simulink model "OscOnly"  (R2022b)
settings: Solver=VariableStepAuto  StartTime=0.0  StopTime=1  RelTol=1e-3
libraries: simulink x1
settings Model: Creator=yoni  LastModifiedBy=yoni

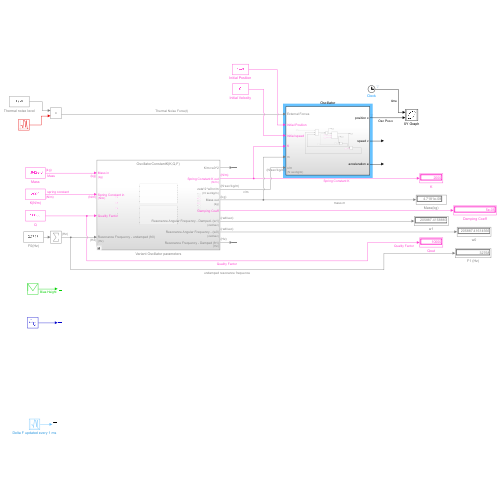
[thumbnail: Simulink's stored preview of the top-level diagram]
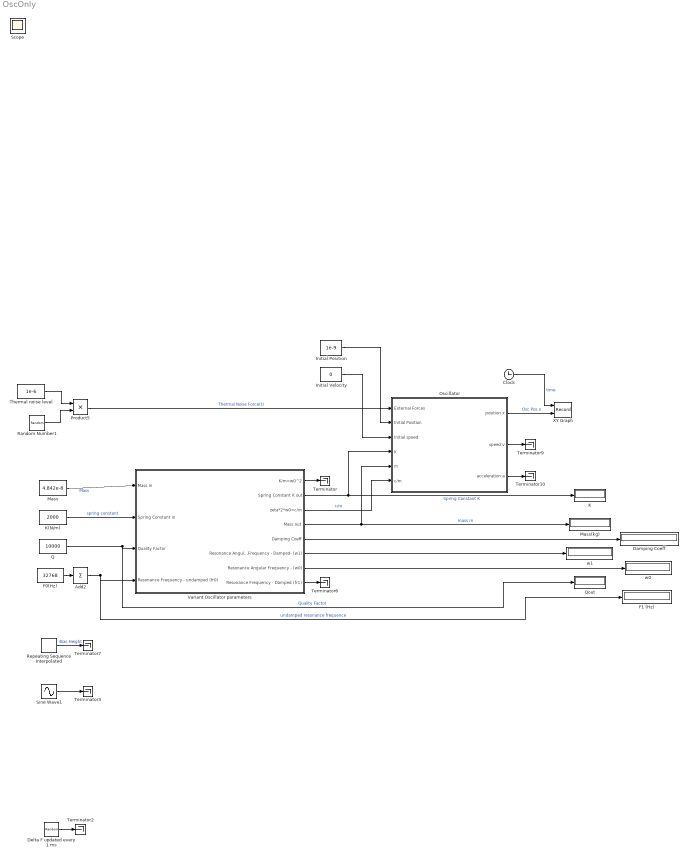
== system OscOnly ==
  Add2 : Sum  Inputs=+
  Clock : Clock
  Damping Coeff : Display
  Delta F updated every 1 ms : RandomNumber  Variance=100  Seed=7546745  SampleTime=1e-3
  F0(Hz) : Constant  Value=32768  SampleTime=-1
  F1 (Hz) : Display
  Initial Position : Constant  Value=1e-9  VectorParams1D=off
  Initial Velocity : Constant  Value=0
  K : Display
  K(N/m) : Constant  Value=2000
  Mass : Constant  Value=4.842e-8
  Mass(kg) : Display
      settings: Format=short_e
  Oscillator : Subsystem
  Product5 : Product
  Q : Constant  Value=10000
  Qout : Display
  Random Number1 : RandomNumber  Seed=4582  SampleTime=10^-8
  Repeating Sequence Interpolated : simulink/Sources/Repeating Sequence Interpolated  OutValues="[25e-10  0.6e-9 25e-10].'"  TimeValues=[0e-3 300e-3 600e-3 ].'  LookUpMeth=Interpolation-Use End Values  tsamp=1e-6  OutMin=[]  OutMax=[]  OutDataTypeStr=double  OutputDataTypeScalingMode=double  OutDataType=fixdt(0,8)  OutScaling=2^-10
  Sine Wave1 : Sin  Amplitude=20  Frequency=5000  Phase=0.0001  SampleTime=10e-6
  Terminator{,2..3,6..7,9..10} (7 alike) : Terminator
  Thermal noise level : Constant  Value=1e-6  VectorParams1D=off  SampleTime=-1
  Variant Oscillator parameters : Subsystem  Variant=on  VariantControlMode=label  LabelModeActiveChoice=OscillatorTypeVar==0  PropagateVariantConditions=on
  XY Graph : Record  FileSettingsInternal="{\"entries\":[{\"content\":{\"excelSettings\":{\"content\":{},\"type\":\"Streamout.ExcelSettings\"}},\"type\":\"Streamout.FileSettingStorage\",\"uuid\":\"efa23a6c-4987-48e8-b3f0-6b34ea382b02\"}],\"packageUris\":[\"http://schema.mathworks.com/mf0/streamout_blocks/R2020a\"],\"version\":\"1.0\"}"  Layout=[1 1]  SignalsInternal="{\"entries\":[{\"content\":{\"signals\":[{\"content\":{\"blockPath\":[\"OscOnly/XY Graph\"],\"channel\":[],\"dimensions\":[1],\"domain\":\"OscOnly/XY Graph\",\"lineColor\":\"#a2142f\",\"plots\":[1],\"port\":1,\"sid\":[\"\"],\"signalID\":691948,\"signalName\":\"time\"},\"type\":\"RecordBlkView.Signal\",\"uuid\":\"d217d77e-fb47-4b7d-b3a2-eb88acfcbc3e\"},{\"content\":{\"blockPath\":[\"OscOnly/XY Graph\"],\"channel\":[],\"dimensions\":[1],\"domain\":\"OscOnly/XY Graph\",\"lineColor\":\"#139fff\",\"plots\":[1],\"port\":2,\"sid\":[\"\"],\"signalID\":691952,\"signalName\":\"Osc Pos x\"},\"type\":\"RecordBlkView.Signal\",\"uuid\":\"5dfddc15-8547-4e19-ad7f-01361fb84854\"}]},\"type\":\"RecordBlkView.InputSignals\",\"uuid\":\"3171f09f-039c-4b49-abe8-6842aea79503\"}],\"packageUris\":[\"http://schema.mathworks.com/mf0/streamout_blocks/R2020a\"],\"version\":\"1.0\"}"  VisualizationBindings="{\"xyplotplugin\":{\"info\":[{\"series\":[{\"bindingParametersList\":[{\"parameter\":\"X-Axis\",\"signalID\":691948,\"signalName\":\"time\"},{\"parameter\":\"Y-Axis\",\"signalID\":691952,\"signalName\":\"Osc Pos x\"}],\"seriesID\":49762}],\"subplotID\":1}]}}"  CompatibilityTag=XY
  w0 : Display
  w1 : Display
  Scope : Scope
  wires:
  Oscillator/2(speed v) -> Terminator9/1
  Initial Velocity/1 -> Oscillator/3(Initial speed)
  Product5/1 -> Oscillator/1(External Forces)  "Thermal Noise Force(t)"
  Variant Oscillator parameters/7(Resonance Angular Frequency - (w0)) -> w0/1
  Oscillator/3(acceleration a) -> Terminator10/1
  Add2/1 -> Variant Oscillator parameters/4(Resonance Frequency - undamped (fr0)), F1 (Hz)/1  "undamped resonance frequence"
  Q/1 -> Variant Oscillator parameters/3(Quality Factor), Qout/1  "Quality Factor"
  Delta F updated every 1 ms/1 -> Terminator2/1
  Variant Oscillator parameters/8(Resonance Frequency - Damped (fr1)) -> Terminator6/1
  Variant Oscillator parameters/6(Resonance Angular Frequency - Damped- (w1)) -> w1/1
  Random Number1/1 -> Product5/2
  Thermal noise level/1 -> Product5/1
  Initial Position/1 -> Oscillator/2(Initial Position)
  Variant Oscillator parameters/3(zeta*2*w0=c/m) -> Oscillator/6(c/m)  "c/m"
  Repeating Sequence Interpolated/1 -> Terminator7/1  "Bias Height"
  Mass/1 -> Variant Oscillator parameters/1(Mass in)  "Mass"
  Variant Oscillator parameters/2(Spring Constant K out) -> K/1, Oscillator/4(K)  "Spring Constant K"
  F0(Hz)/1 -> Add2/1
  Variant Oscillator parameters/4(Mass out) -> Mass(kg)/1, Oscillator/5(m)  "mass m"
  K(N/m)/1 -> Variant Oscillator parameters/2(Spring Constant in)  "spring constant"
  Variant Oscillator parameters/1(K/m=w0^2) -> Terminator/1
  Variant Oscillator parameters/5(Damping Coeff) -> Damping Coeff/1
  Sine Wave1/1 -> Terminator3/1
  Oscillator/1(" position x") -> XY Graph/2  "Osc Pos x"
  Clock/1 -> XY Graph/1  "time"

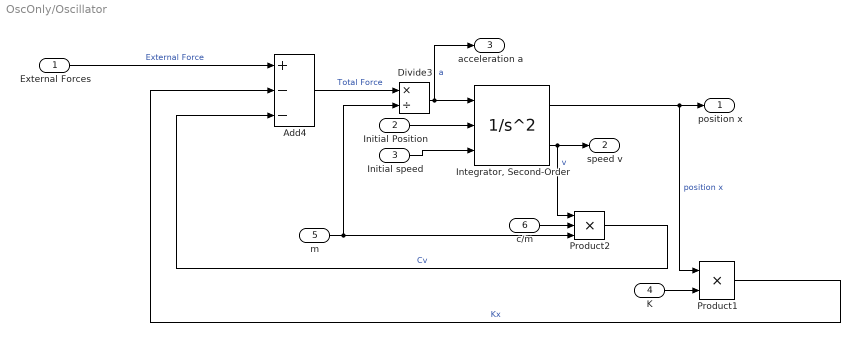
== system OscOnly/Oscillator ==
  External Forces : Inport
  Initial Position : Inport  Port=2
  Initial speed : Inport  Port=3
  K : Inport  Port=4
  m : Inport  Port=5
  c/m : Inport  Port=6  Unit=N*sec/kg/m
  Add4 : Sum  Inputs=+--
  Divide3 : Product  Inputs=*/
  "Integrator, Second-Order" : SecondOrderIntegrator  ICSourceX=external  LimitX=on  UpperLimitX=0.01  LowerLimitX=-0.01  ICSourceDXDT=external
  Product1 : Product
  Product2 : Product  Inputs=3
  " position x" : Outport
  speed v : Outport  Port=2
  acceleration a : Outport  Port=3
  wires:
  Divide3/1 -> "Integrator, Second-Order"/1, acceleration a/1  "a"
  m/1 -> Divide3/2, Product2/3
  Product1/1 -> Add4/2  "Kx"
  c/m/1 -> Product2/2
  Initial speed/1 -> "Integrator, Second-Order"/3
  Add4/1 -> Divide3/1  "Total Force"
  External Forces/1 -> Add4/1  "External Force"
  K/1 -> Product1/2
  "Integrator, Second-Order"/2 -> speed v/1, Product2/1  "v"
  Product2/1 -> Add4/3  "Cv"
  "Integrator, Second-Order"/1 -> Product1/1, " position x"/1  "position x"
  Initial Position/1 -> "Integrator, Second-Order"/2

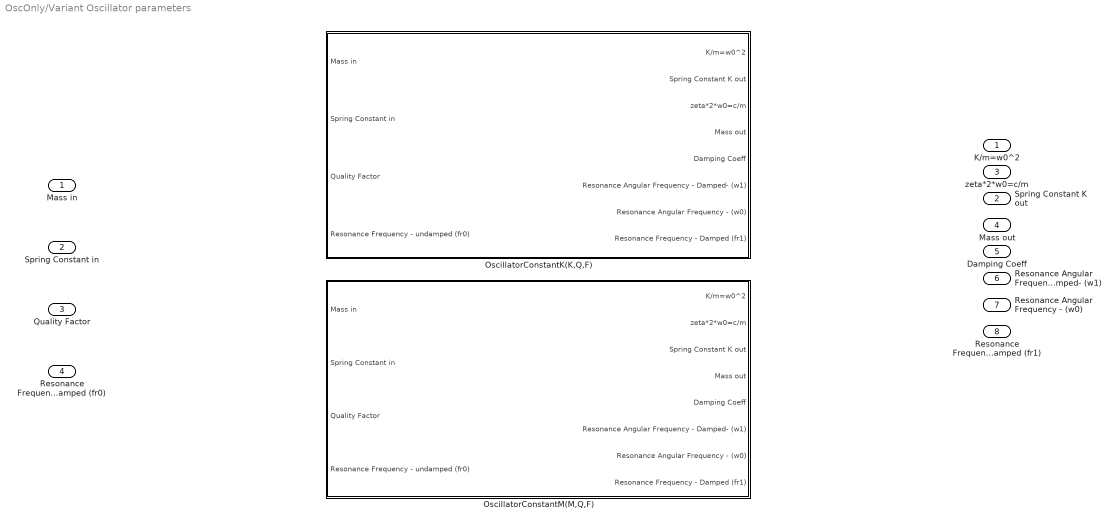
== system OscOnly/Variant Oscillator parameters ==
  Mass in : Inport  Unit=kg
  Spring Constant in : Inport  Port=2  Unit=N/m
  Quality Factor : Inport  Port=3
  Resonance Frequency - undamped (fr0) : Inport  Port=4  Unit=Hz
  OscillatorConstantK(K,Q,F) : Subsystem  VariantControl=OscillatorTypeVar==0
  OscillatorConstantM(M,Q,F) : Subsystem  VariantControl=OscillatorTypeVar==1
  K/m=w0^2 : Outport  VectorParamsAs1DForOutWhenUnconnected=off
  Spring Constant K out : Outport  Port=2  Unit=N/m  VectorParamsAs1DForOutWhenUnconnected=off
  zeta*2*w0=c/m : Outport  Port=3  Unit=N*sec/kg/m  VectorParamsAs1DForOutWhenUnconnected=off
  Mass out : Outport  Port=4  Unit=kg  VectorParamsAs1DForOutWhenUnconnected=off
  Damping Coeff : Outport  Port=5  VectorParamsAs1DForOutWhenUnconnected=off
  Resonance Angular Frequency - Damped- (w1) : Outport  Port=6  Unit=rad/sec  VectorParamsAs1DForOutWhenUnconnected=off
  Resonance Angular Frequency - (w0) : Outport  Port=7  Unit=rad/sec  VectorParamsAs1DForOutWhenUnconnected=off
  Resonance Frequency - Damped (fr1) : Outport  Port=8  Unit=Hz  VectorParamsAs1DForOutWhenUnconnected=off

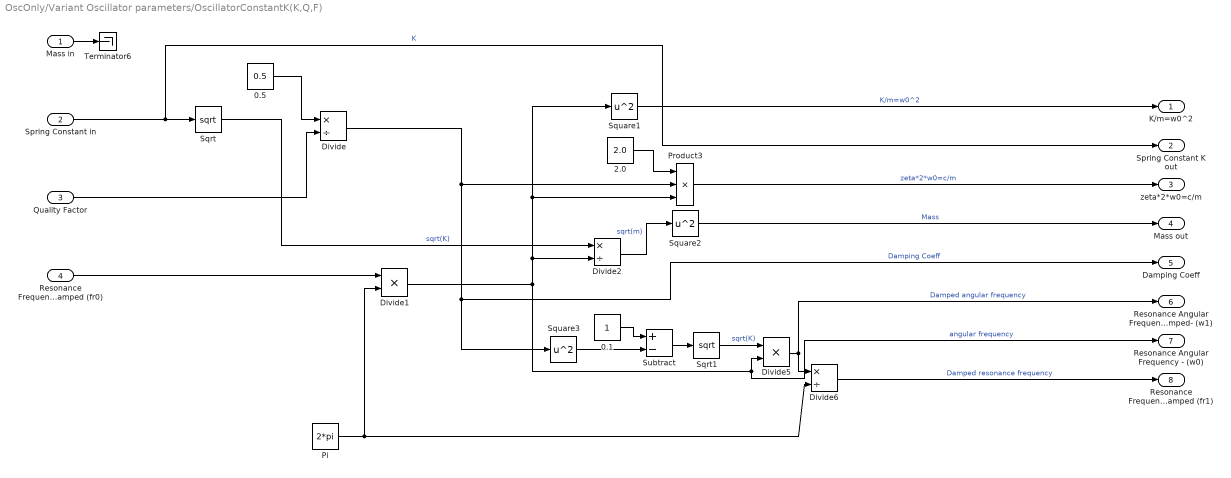
== system OscOnly/Variant Oscillator parameters/OscillatorConstantK(K,Q,F) ==
  Mass in : Inport  Unit=kg
  Spring Constant in : Inport  Port=2  Unit=N/m
  Quality Factor : Inport  Port=3
  Resonance Frequency - undamped (fr0) : Inport  Port=4  Unit=Hz
  0.1 : Constant
  0.5 : Constant  Value=0.5
  2.0 : Constant  Value=2.0
  Divide : Product  Inputs=*/
  Divide1 : Product  Inputs=**
  Divide2 : Product  Inputs=*/
  Divide5 : Product  Inputs=**
  Divide6 : Product  Inputs=*/
  Pi : Constant  Value=2*pi  OutDataTypeStr=Inherit: Inherit via back propagation
  Product3 : Product  Inputs=3
  Sqrt : Sqrt
  Sqrt1 : Sqrt
  Square1 : Math  Operator=square  SignedPower=on
  Square2 : Math  Operator=square  SignedPower=on
  Square3 : Math  Operator=square  SignedPower=on
  Subtract : Sum  Inputs=+-
  Terminator6 : Terminator
  K/m=w0^2 : Outport  VectorParamsAs1DForOutWhenUnconnected=off
  Spring Constant K out : Outport  Port=2  Unit=N/m  VectorParamsAs1DForOutWhenUnconnected=off
  zeta*2*w0=c/m : Outport  Port=3  VectorParamsAs1DForOutWhenUnconnected=off
  Mass out : Outport  Port=4  Unit=kg  VectorParamsAs1DForOutWhenUnconnected=off
  Damping Coeff : Outport  Port=5  VectorParamsAs1DForOutWhenUnconnected=off
  Resonance Angular Frequency - Damped- (w1) : Outport  Port=6  Unit=rad/sec  VectorParamsAs1DForOutWhenUnconnected=off
  Resonance Angular Frequency - (w0) : Outport  Port=7  Unit=rad/sec  VectorParamsAs1DForOutWhenUnconnected=off
  Resonance Frequency - Damped (fr1) : Outport  Port=8  Unit=Hz  VectorParamsAs1DForOutWhenUnconnected=off
  wires:
  Divide1/1 -> Square1/1, Product3/3, Divide2/2, Divide5/2, Resonance Angular Frequency - (w0)/1  "angular frequency"
  Divide5/1 -> Divide6/1, Resonance Angular Frequency - Damped- (w1)/1  "Damped angular frequency"
  0.5/1 -> Divide/1
  Divide2/1 -> Square2/1  "sqrt(m)"
  0.1/1 -> Subtract/1
  Divide/1 -> Square3/1, Damping Coeff/1, Product3/2  "Damping Coeff"
  Square3/1 -> Subtract/2
  Sqrt1/1 -> Divide5/1  "sqrt(K)"
  Subtract/1 -> Sqrt1/1
  Sqrt/1 -> Divide2/1  "sqrt(K)"
  Square1/1 -> K/m=w0^2/1  "K/m=w0^2"
  Pi/1 -> Divide1/2, Divide6/2
  2.0/1 -> Product3/1
  Resonance Frequency - undamped (fr0)/1 -> Divide1/1
  Quality Factor/1 -> Divide/2
  Product3/1 -> zeta*2*w0=c/m/1  "zeta*2*w0=c/m"
  Divide6/1 -> Resonance Frequency - Damped (fr1)/1  "Damped resonance frequency"
  Square2/1 -> Mass out/1  "Mass"
  Spring Constant in/1 -> Spring Constant K out/1, Sqrt/1  "K"
  Mass in/1 -> Terminator6/1

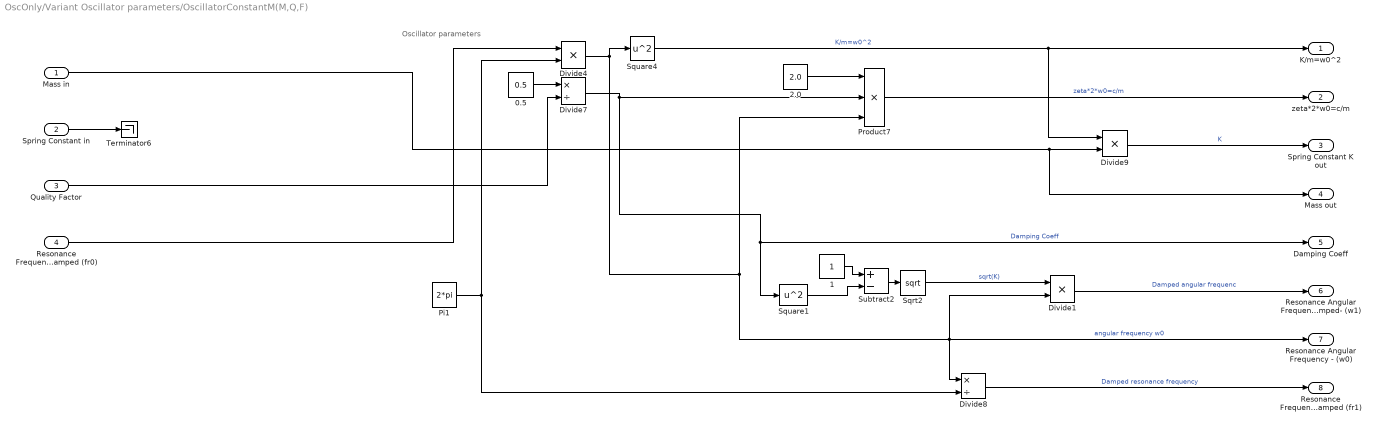
== system OscOnly/Variant Oscillator parameters/OscillatorConstantM(M,Q,F) ==
  note: Oscillator parameters
  Mass in : Inport  Unit=kg
  Spring Constant in : Inport  Port=2  Unit=N/m
  Quality Factor : Inport  Port=3
  Resonance Frequency - undamped (fr0) : Inport  Port=4  Unit=Hz
  0.5 : Constant  Value=0.5
  1 : Constant
  2.0 : Constant  Value=2.0
  Divide1 : Product  Inputs=**
  Divide4 : Product  Inputs=**
  Divide7 : Product  Inputs=*/
  Divide8 : Product  Inputs=*/
  Divide9 : Product  Inputs=**
  Pi1 : Constant  Value=2*pi  OutDataTypeStr=Inherit: Inherit via back propagation
  Product7 : Product  Inputs=3
  Sqrt2 : Sqrt
  Square1 : Math  Operator=square  SignedPower=on
  Square4 : Math  Operator=square  SignedPower=on
  Subtract2 : Sum  Inputs=+-
  Terminator6 : Terminator
  K/m=w0^2 : Outport  Unit=N/(kg*m)  VectorParamsAs1DForOutWhenUnconnected=off
  zeta*2*w0=c/m : Outport  Port=2  Unit=N*sec/kg/m  VectorParamsAs1DForOutWhenUnconnected=off
  Spring Constant K out : Outport  Port=3  Unit=N/m  VectorParamsAs1DForOutWhenUnconnected=off
  Mass out : Outport  Port=4  Unit=kg  VectorParamsAs1DForOutWhenUnconnected=off
  Damping Coeff : Outport  Port=5  VectorParamsAs1DForOutWhenUnconnected=off
  Resonance Angular Frequency - Damped- (w1) : Outport  Port=6  Unit=rad/sec  VectorParamsAs1DForOutWhenUnconnected=off
  Resonance Angular Frequency - (w0) : Outport  Port=7  Unit=rad/sec  VectorParamsAs1DForOutWhenUnconnected=off
  Resonance Frequency - Damped (fr1) : Outport  Port=8  Unit=Hz  VectorParamsAs1DForOutWhenUnconnected=off
  wires:
  Resonance Frequency - undamped (fr0)/1 -> Divide4/1
  Sqrt2/1 -> Divide1/1  "sqrt(K)"
  Square4/1 -> Divide9/1, K/m=w0^2/1  "K/m=w0^2"
  Pi1/1 -> Divide4/2, Divide8/2
  Divide7/1 -> Square1/1, Damping Coeff/1, Product7/2  "Damping Coeff"
  Divide4/1 -> Square4/1, Product7/3, Divide1/2, Divide8/1, Resonance Angular Frequency - (w0)/1  "angular frequency w0"
  Divide1/1 -> Resonance Angular Frequency - Damped- (w1)/1  "Damped angular frequenc"
  2.0/1 -> Product7/1
  Divide8/1 -> Resonance Frequency - Damped (fr1)/1  "Damped resonance frequency"
  Subtract2/1 -> Sqrt2/1
  Square1/1 -> Subtract2/2
  0.5/1 -> Divide7/1
  1/1 -> Subtract2/1
  Mass in/1 -> Mass out/1, Divide9/2
  Divide9/1 -> Spring Constant K out/1  "K"
  Product7/1 -> zeta*2*w0=c/m/1  "zeta*2*w0=c/m"
  Quality Factor/1 -> Divide7/2
  Spring Constant in/1 -> Terminator6/1
